simulink model "p5d"  (R2017a)
settings: Solver=ode45  StartTime=0.0  StopTime=inf  RelTol=1e-3  EnableMultiTasking=on
values from neighbouring files (symbols this model uses):
  K_pd = 0.8363    [p5_init.m]
  T_d = T    [p5_init.m]
  T_f = 8.3909    [p5_init.m]
  Ts = 1/Fs    (= 0.1)    [p5_init.m]
libraries: simulink_extras x6, simulink x2
settings Model: Creator=markh  LastModifiedBy=arefv
settings DataIOCC: LimitDataPoints=on  SaveFormat=Array  SignalLoggingSaveFormat=ModelDataLogs  SignalLoggingName=sigsOut
settings OptimizationCC: InitFltsAndDblsToZero=on  LifeSpan=inf
settings DebuggingCC: SaveWithParameterizedLinksMsg=none  UnderspecifiedInitializationDetection=Classic  MergeDetectMultiDrivingBlocksExec=none  SignalResolutionControl=TryResolveAllWithWarning  MultiTaskDSMMsg=warning  MultiTaskCondExecSysMsg=none  FcnCallInpInsideContextMsg=warning  StateNameClashWarn=warning  SFUnexpectedBacktrackingDiag=warning  SFNoUnconditionalDefaultTransitionDiag=warning  SFExecutionAtInitializationDiag=none
settings HardwareCC: ProdBitPerPointer=32  ProdBitPerSizeT=32  ProdBitPerPtrDiffT=32  ProdLargestAtomicFloat=None  ProdIntDivRoundTo=Undefined  ProdEndianess=Unspecified  ProdWordSize=32  ProdHWDeviceType=32-bit Generic  TargetBitPerPointer=64  TargetBitPerSizeT=64  TargetBitPerPtrDiffT=64  TargetLongLongMode=on  TargetIntDivRoundTo=Zero  TargetEndianess=LittleEndian  TargetWordSize=64  TargetHWDeviceType=MATLAB Host  ProdEqTarget=off
settings ModelReferenceCC: PropagateSignalLabelsOutOfModel=off
settings GRTTargetCC: TargetFcnLib=ansi_tfl_tmw.mat  TargetLangStandard=C89/C90 (ANSI)  GeneratePreprocessorConditionals=Disable all  CombineOutputUpdateFcns=off  GRTInterface=on
settings ConfigComp: CovMetricSettings=dw  CovHtmlReporting=on  CovSaveCumulativeToWorkspaceVar=on  CovSaveSingleToWorkspaceVar=on  CovExternalEMLEnable=off

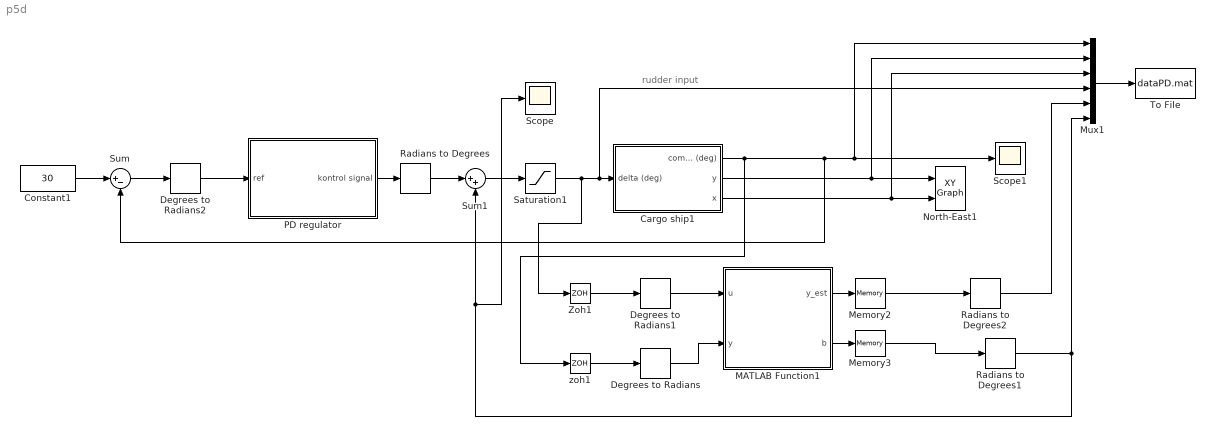
== system p5d ==
  note: rudder input
  Cargo ship1 : Subsystem  mask(Simple shipmodel for a cargo ship){noise=on, current=on, logic=off}
      mask prompts: noise "measurement noise"; logic "waves"
      mask help:
      | Measurement noise:
      | 	checked = noise on
      | 	unchecked = noise off
      |
      | Current:
      | 	checked = current on
      | 	unchecked = current off
      |
      | Waves:
      | 	checked = waves on
      | 	unchecked = waves off
      |
      | Author: Jørgen Spjøtvold, 9/10-2003
      | TTK 4115 Linear system theory.
      | Modified by Jostein Bakkeheim 26/10-2006
  Constant1 : Constant  Value=30
  Degrees to Radians : simulink_extras/Transformations/Degrees to Radians
  Degrees to Radians1 : simulink_extras/Transformations/Degrees to Radians
  Degrees to Radians2 : simulink_extras/Transformations/Degrees to Radians
  MATLAB Function1 : MATLAB Function  TreatAsAtomicUnit=on
  Memory2 : Memory
  Memory3 : Memory
  Mux1 : Mux  Inputs=6
  North-East1 : simulink/Sinks/XY Graph  xmin=-5000  xmax=5000  ymin=-5000  ymax=5000  st=-1
  "PD regulator " : Subsystem
  Radians to Degrees : simulink_extras/Transformations/Radians to Degrees
  Radians to Degrees1 : simulink_extras/Transformations/Radians to Degrees
  Radians to Degrees2 : simulink_extras/Transformations/Radians to Degrees
  Saturation1 : Saturate  UpperLimit=35  LowerLimit=-35
  Scope : Scope
  Scope1 : Scope
  Sum : Sum  Inputs=|+-
  Sum1 : Sum  Inputs=|++
  To File : ToFile  Filename=dataPD.mat  MatrixName=dataPD
  Zoh1 : ZeroOrderHold  SampleTime=Ts
  zoh1 : ZeroOrderHold  SampleTime=Ts
  wires:
  MATLAB Function1/2(b) -> Memory3/1
  MATLAB Function1/1(y_est) -> Memory2/1
  Saturation1/1 -> Zoh1/1, Mux1/4, Cargo ship1/1(delta (deg))
  zoh1/1 -> Degrees to Radians/1
  Cargo ship1/2(y) -> Mux1/2, North-East1/1
  Cargo ship1/1(compass (deg)) -> zoh1/1, Sum/2, Scope1/1, Mux1/1
  Memory3/1 -> Radians to Degrees1/1
  Memory2/1 -> Radians to Degrees2/1
  Cargo ship1/3(x) -> Mux1/3, North-East1/2
  Constant1/1 -> Sum/1
  Zoh1/1 -> Degrees to Radians1/1
  Sum1/1 -> Saturation1/1
  Degrees to Radians2/1 -> "PD regulator "/1(ref)
  "PD regulator "/1("kontrol signal ") -> Radians to Degrees/1
  Radians to Degrees/1 -> Sum1/1
  Sum/1 -> Degrees to Radians2/1
  Mux1/1 -> To File/1
  Degrees to Radians/1 -> MATLAB Function1/2(y)
  Degrees to Radians1/1 -> MATLAB Function1/1(u)
  Radians to Degrees2/1 -> Mux1/5
  Radians to Degrees1/1 -> Mux1/6, Scope/1, Sum1/2

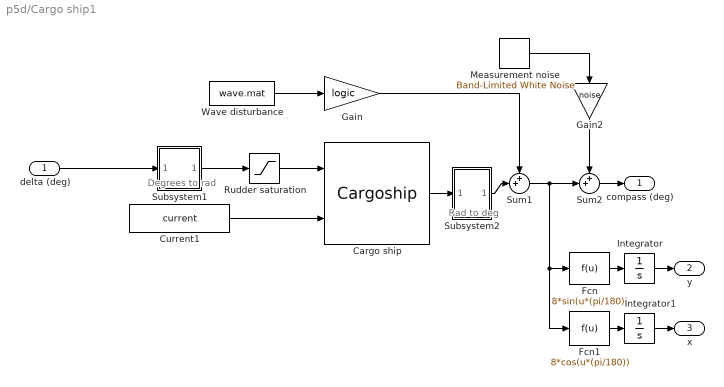
== system p5d/Cargo ship1 ==
  note: Degrees to rad
  note: Rad to deg
  delta (deg) : Inport
  Cargo ship : S-Function  FunctionName=Cargoship  SFunctionDeploymentMode=off  EnableBusSupport=off  mask(Cargo ship){}
      mask help:
      | S-function which simulates a cargo ship.
      |
      | Author: Jørgen Spjøtvold
      | 20.10-2003
      | Modified by Jostein Bakkeheim 27.10.2006
  Current1 : Constant  Value=current
  Fcn : Fcn  Expr=8*sin(u*(pi/180))
  Fcn1 : Fcn  Expr=8*cos(u*(pi/180))
  Gain : Gain  Gain=logic  SaturateOnIntegerOverflow=on  OutDataTypeStr=Inherit: Same as input  ParamDataTypeStr=Inherit: Same as input
  Gain2 : Gain  Gain=noise  SaturateOnIntegerOverflow=on  OutDataTypeStr=Inherit: Same as input  ParamDataTypeStr=Inherit: Same as input
  Integrator : Integrator
  Integrator1 : Integrator
  Measurement noise : simulink/Sources/Band-Limited White Noise  Cov=[0.001]  Ts=.5  seed=[23341]
  Rudder saturation : Saturate  UpperLimit=45*(pi/180)  LowerLimit=-45*(pi/180)
  Subsystem1 : Subsystem  mask(degrees to radians){}
      mask help: Converts degrees to radians
      mask Display: fprintf('D2R');
  Subsystem2 : Subsystem  mask(radians to degrees){}
      mask help: Converts radians to degrees
      mask Display: fprintf('R2D');
  Sum1 : Sum  Inputs=++|  SaturateOnIntegerOverflow=on
  Sum2 : Sum  Inputs=++|  SaturateOnIntegerOverflow=on
  Wave disturbance : FromFile  FileName=wave.mat  SampleTime=0
  compass (deg) : Outport
  y : Outport  Port=2
  x : Outport  Port=3
  wires:
  delta (deg)/1 -> Subsystem1/1(In1)
  Fcn/1 -> Integrator/1
  Integrator/1 -> y/1
  Fcn1/1 -> Integrator1/1
  Integrator1/1 -> x/1
  Wave disturbance/1 -> Gain/1
  Subsystem2/1(Out1) -> Sum1/2
  Gain/1 -> Sum1/1
  Sum1/1 -> Fcn/1, Fcn1/1, Sum2/2
  Cargo ship/1 -> Subsystem2/1(In1)
  Subsystem1/1(Out1) -> Rudder saturation/1
  Rudder saturation/1 -> Cargo ship/1
  Sum2/1 -> compass (deg)/1
  Measurement noise/1 -> Gain2/1
  Gain2/1 -> Sum2/1
  Current1/1 -> Cargo ship/2

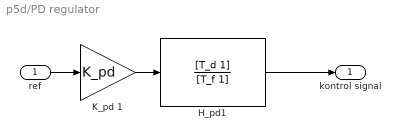
== system p5d/PD regulator  ==
  ref : Inport
  H_pd1 : TransferFcn  Numerator=[T_d 1]  Denominator=[T_f 1]
  K_pd 1 : Gain  Gain=K_pd
  "kontrol signal " : Outport
  wires:
  H_pd1/1 -> "kontrol signal "/1
  ref/1 -> K_pd 1/1
  K_pd 1/1 -> H_pd1/1

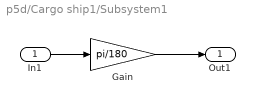
== system p5d/Cargo ship1/Subsystem1 ==
  In1 : Inport
  Gain : Gain  Gain=pi/180  SaturateOnIntegerOverflow=on  OutDataTypeStr=Inherit: Same as input  ParamDataTypeStr=Inherit: Same as input
  Out1 : Outport
  wires:
  Gain/1 -> Out1/1
  In1/1 -> Gain/1

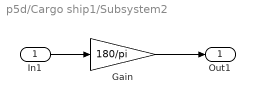
== system p5d/Cargo ship1/Subsystem2 ==
  In1 : Inport
  Gain : Gain  Gain=180/pi  SaturateOnIntegerOverflow=on  OutDataTypeStr=Inherit: Same as input  ParamDataTypeStr=Inherit: Same as input
  Out1 : Outport
  wires:
  Gain/1 -> Out1/1
  In1/1 -> Gain/1

== matlab function p5d/MATLAB Function1 ==
  data: u input; y_est output; y input; b output; ks parameter
function [y_est,b] = kalman(u,y,ks)
persistent init x_pri P_pri Ad Bd C Ed Q I R 

if isempty(init)
    %Initializing constants
    Ad=ks.Ad;   Bd=ks.Bd;   C=ks.C; Ed=ks.Ed;
    I=ks.I; R=ks.R; Q=ks.Q; 
    % Initializing first step
    x_pri = ks.x0_pri;
    P_pri = ks.P0_pri;
    % Making sure initializing only once
    init = 1;
end
% Calculating Kalman gain
K = P_pri*C'*inv(C*P_pri*C'+R);

% Updating the Kalman filter
x_post = x_pri+K*(y-C*x_pri);           % Update estimate with measurement
P_post = (I-K*C)*P_pri*(I-K*C)'+K*R*K'; % Update error covariance matrix

%Project ahead
x_pri = Ad*x_post+Bd*u;
P_pri = Ad*P_post*Ad'+Ed*Q*Ed';

% Setting the output
y_est = x_post(3);     b = x_post(5);
end
